simulink model "sampleModel188"  (R2021b)
settings: Solver=VariableStepAuto  StartTime=0.0  StopTime=10.0  RelTol=1e-3
libraries: simulink x11, slpidlib x1
settings Model: Creator=user  LastModifiedBy=user

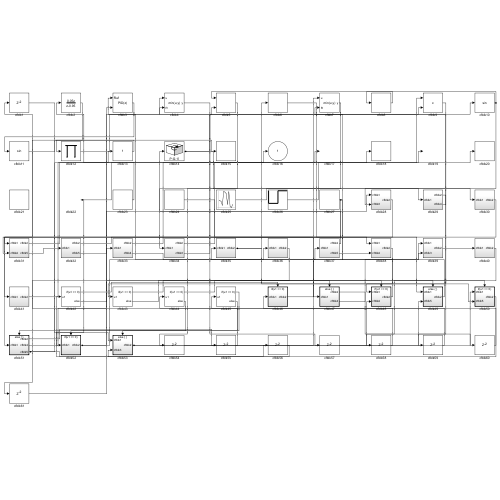
[thumbnail: Simulink's stored preview of the top-level diagram]
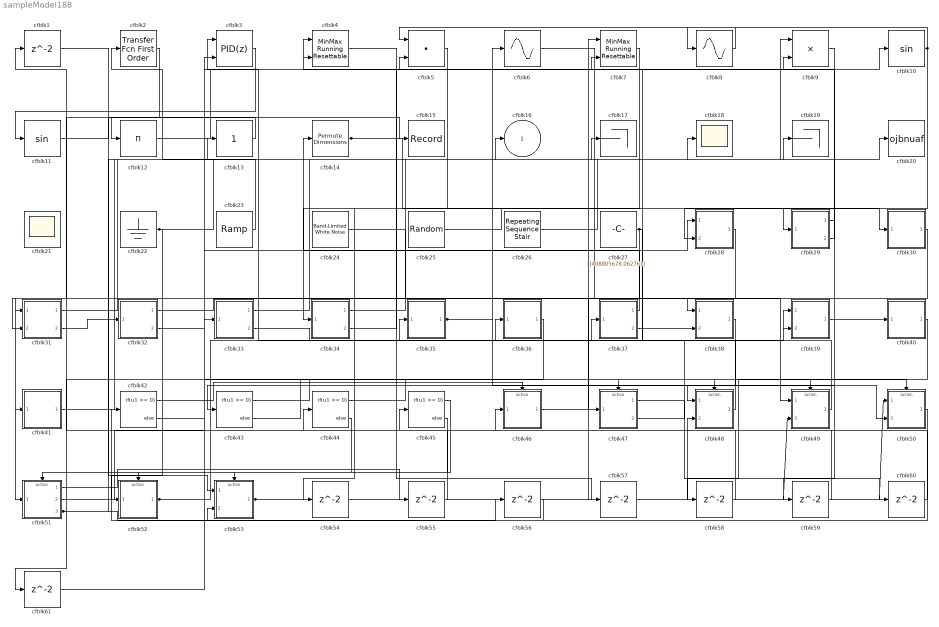
== system sampleModel188 ==
  cfblk{1,54..61} (9 alike) : Delay  SampleTime=1
  cfblk10 : Trigonometry
  cfblk11 : Trigonometry
  cfblk12 : Product  Inputs=*
  cfblk13 : simulink/Math Operations/Slider Gain  gain=1  low=0  high=2
  cfblk14 : PermuteDimensions
  cfblk15 : Record  FileSettingsInternal="{\"entries\":[{\"content\":{\"excelSettings\":{\"content\":{},\"type\":\"Streamout.ExcelSettings\"}},\"type\":\"Streamout.FileSettingStorage\",\"uuid\":\"ca993f84-a60c-403e-8350-93dc5c48e853\"}],\"packageUris\":[\"http://schema.mathworks.com/mf0/streamout_blocks/R2020a\"],\"version\":\"1.0\"}"  SignalsInternal="{\"entries\":[{\"content\":{\"signals\":[{\"content\":{\"blockPath\":[\"sampleModel188/cfblk15\"],\"channel\":[],\"dimensions\":[1,1],\"domain\":\"sampleModel188/cfblk15\",\"lineColor\":\"#139fff\",\"plots\":[1],\"port\":1,\"sid\":[\"\"],\"signalID\":7064,\"signalName\":\"cfblk11\"},\"type\":\"RecordBlkView.Signal\",\"uuid\":\"ba3ac5e5-cf71-48a5-8aa6-1fcd734a01e5\"}]},\"type\":\"RecordBlkView.InputSignals\",\"uuid\":\"2d8e7e94-0d17-40cb-8f9e-080a064f809d\"}],\"packageUris\":[\"http://schema.mathworks.com/mf0/streamout_blocks/R2020a\"],\"version\":\"1.0\"}"  VisualizationBindings="{\"sparklinesplugin\":{\"info\":[{\"bindingParametersList\":[],\"subplotID\":1}]}}"
  cfblk17 : Terminator
  cfblk18 : Scope
  cfblk19 : Terminator
  cfblk2 : simulink/Discrete/Transfer Fcn First Order  PoleZ=0.95  ICPrevOutput=0.0  DoSatur=off
  cfblk20 : ToWorkspace  VariableName=ojbnuaf  SaveFormat=Timeseries  SampleTime=-1
  cfblk21 : Scope
      settings: Floating=on
  cfblk22 : Ground
  cfblk23 : simulink/Sources/Ramp  slope=[6918.058367]  start=[43.830131]  InitialOutput=[-707195.429507]
  cfblk24 : simulink/Sources/Band-Limited White Noise  Cov=[2157080440.505384]  Ts=0.1  seed=[4930132520.000000]
  cfblk25 : RandomNumber  Mean=[-27753.868403]  Variance=[17619.578113]  Seed=[28560651.000000]  SampleTime=0.1
  cfblk26 : simulink/Sources/Repeating Sequence Stair  OutValues=[-496034706.787339, -122048597.583753]  tsamp=-1  OutMin=[]  OutMax=[]  OutDataTypeStr=double  OutputDataTypeScalingMode=double  OutDataType=fixdt(0,8)  ConRadixGroup=Best Precision: Vector-wise  OutScaling=2^-12
  cfblk27 : Constant  Value=[408805678.062761]  SampleTime=1
  cfblk28 : Subsystem
  cfblk29 : Subsystem
  cfblk3 : slpidlib/PID Controller (2DOF)  Controller=PID  Form=Parallel  TimeDomain=Discrete-time  UseExternalTs=off  SampleTime=1  IntegratorMethod=Forward Euler  FilterMethod=Forward Euler  ControllerParametersSource=internal  P=1  I=1  D=0  UseFilter=on  N=100  b=1  c=1  TunerSelectOption=Transfer Function Based (PID Tuner App)  InitialConditionSource=internal  InitialConditionForIntegrator=0  InitialConditionForFilter=0  DifferentiatorICPrevScaledInput=0  ExternalReset=none  TrackingMode=off  Kt=1  LimitOutput=off  SatLimitsSource=internal  UpperSaturationLimit=inf  LowerSaturationLimit=-inf  LinearizeAsGain=off  AntiWindupMode=none  Kb=1  POutMin=[]  POutMax=[]  IOutMin=[]  IOutMax=[]  DOutMin=[]  DOutMax=[]  NOutMin=[]  NOutMax=[]  bOutMin=[]  bOutMax=[]  cOutMin=[]  cOutMax=[]  SumOutMin=[]  SumOutMax=[]  SaturationOutMin=[]  SaturationOutMax=[]  PParamMin=[]  PParamMax=[]  IParamMin=[]  IParamMax=[]  DParamMin=[]  DParamMax=[]  NParamMin=[]  NParamMax=[]  bParamMin=[]  bParamMax=[]  cParamMin=[]  cParamMax=[]  KbParamMin=[]  KbParamMax=[]  KtParamMin=[]  KtParamMax=[]  KbOutMin=[]  KbOutMax=[]  KtOutMin=[]  KtOutMax=[]  IntegratorOutMin=[]  IntegratorOutMax=[]  FilterOutMin=[]  FilterOutMax=[]  SumI1OutMin=[]  SumI1OutMax=[]  SumI2OutMin=[]  SumI2OutMax=[]  SumI3OutMin=[]  SumI3OutMax=[]  SumI4OutMin=[]  SumI4OutMax=[]  SumDOutMin=[]  SumDOutMax=[]  Sum1OutMin=[]  Sum1OutMax=[]  Sum2OutMin=[]  Sum2OutMax=[]  Sum3OutMin=[]  Sum3OutMax=[]  DifferentiatorOutMin=[]  DifferentiatorOutMax=[]  FilterDiffOutCoefMin=[]  FilterDiffOutCoefMax=[]  ReciprocalOutMin=[]  ReciprocalOutMax=[]  SumDenOutMin=[]  SumDenOutMax=[]  SumNumOutMin=[]  SumNumOutMax=[]  DivideOutMin=[]  DivideOutMax=[]  UdiffTsProdOutMin=[]  UdiffTsProdOutMax=[]  NTsProdOutMin=[]  NTsProdOutMax=[]  UintegralTsProdOutMin=[]  UintegralTsProdOutMax=[]  UngainTsProdOutMin=[]  UngainTsProdOutMax=[]  IntegratorContinuousStateAttributes=''  IntegratorStateMustResolveToSignalObject=off  IntegratorRTWStateStorageClass=Auto  FilterContinuousStateAttributes=''  FilterStateMustResolveToSignalObject=off  FilterRTWStateStorageClass=Auto  ParallelPVariant=InternalParameters  IdealPVariant=Disabled  IVariant=InternalParameters  DVariant=InternalParameters  bVariant=InternalParameters  cVariant=InternalParameters  IntegratorVariant=Discrete  SatVariant=Disabled  AWVariant=Passthrough  PCopyVariant=Disabled  TRVariant=Disabled  FdbkBlocksVariant=Forward  IdealPFdbkVariant=Disabled  SatFdbkVariant=Disabled  DerivativeFilterVariant=ForwardEulerFilter  NVariant=InternalParameters  NCopyVariant=Disabled  FilterICVariant=InternalICsFilter  IntegratorICVariant=InternalICs  ExternalResetVariant=Disabled  TRSumVariant=Passthrough  SumFdbkVariant=Disabled  SumVariant=Sum_PID  TsampFilterVariant=InternalTs  TsampNgainVariant=Passthrough  TsampIntegralVariant=Passthrough  ExternalSaturationOutDataTypeStr=Inherit: Same as second input
      settings: SourceProductBaseCode=SL
  cfblk30 : Subsystem
  cfblk31 : Subsystem
  cfblk32 : Subsystem
  cfblk33 : Subsystem
  cfblk34 : Subsystem
  cfblk35 : Subsystem
  cfblk36 : Subsystem
  cfblk37 : Subsystem
  cfblk38 : Subsystem
  cfblk39 : Subsystem
  cfblk4 : simulink/Math Operations/MinMax Running Resettable  Function=min  vinit=0.0
  cfblk40 : Subsystem
  cfblk41 : Subsystem
  cfblk{42..45} (4 alike) : If  IfExpression=u1 >= 0  SampleTime=1
  cfblk46 : Subsystem  TreatAsAtomicUnit=on
  cfblk47 : Subsystem  TreatAsAtomicUnit=on
  cfblk48 : Subsystem  TreatAsAtomicUnit=on
  cfblk49 : Subsystem  TreatAsAtomicUnit=on
  cfblk5 : DotProduct  InputSameDT=on  OutDataTypeStr=Inherit: Inherit via internal rule
  cfblk50 : Subsystem  TreatAsAtomicUnit=on
  cfblk51 : Subsystem  TreatAsAtomicUnit=on
  cfblk52 : Subsystem  TreatAsAtomicUnit=on
  cfblk53 : Subsystem  TreatAsAtomicUnit=on
  cfblk6 : Sin  TimeSource=Use external signal  SampleTime=0
  cfblk7 : simulink/Math Operations/MinMax Running Resettable  Function=min  vinit=0.0
  cfblk8 : Sin  TimeSource=Use external signal  SampleTime=0
  cfblk9 : Product
  cfblk16 : Outport
  wires:
  cfblk29/1(cfblk2) -> cfblk48/1(cfblk1)
  cfblk41/1(cfblk2) -> cfblk19/1
  cfblk13/1 -> cfblk12/1
  cfblk3/1 -> cfblk11/1
  cfblk37/1(cfblk2) -> cfblk14/1
  cfblk27/1 -> cfblk35/1(cfblk1), cfblk31/2(cfblk4)
  cfblk12/1 -> cfblk4/1
  cfblk7/1 -> cfblk34/1(cfblk1)
  cfblk52/1(cfblk2) -> cfblk37/1(cfblk1), cfblk5/2
  cfblk33/1(cfblk2) -> cfblk16/1
  cfblk38/1(cfblk2) -> cfblk43/1
  cfblk26/1 -> cfblk18/1
  cfblk24/1 -> cfblk47/1(cfblk1)
  cfblk14/1 -> cfblk29/1(cfblk1), cfblk9/2
  cfblk35/1(cfblk2) -> cfblk6/1, cfblk50/2(cfblk5)
  cfblk25/1 -> cfblk30/1(cfblk1)
  cfblk33/2(cfblk4) -> cfblk36/1(cfblk1)
  cfblk23/1 -> cfblk2/1
  cfblk28/1(cfblk2) -> cfblk51/1(cfblk1)
  cfblk47/2(cfblk4) -> cfblk39/1(cfblk1)
  cfblk46/1(cfblk2) -> cfblk39/2(cfblk3)
  cfblk6/1 -> cfblk49/1(cfblk1)
  cfblk31/1(cfblk2) -> cfblk20/1
  cfblk29/2(cfblk4) -> cfblk4/2
  cfblk34/1(cfblk2) -> cfblk17/1
  cfblk32/1(cfblk2) -> cfblk38/1(cfblk1)
  cfblk10/1 -> cfblk8/1, cfblk28/2(cfblk3)
  cfblk50/1(cfblk2) -> cfblk42/1
  cfblk31/2(cfblk5) -> cfblk32/1(cfblk1)
  cfblk48/1(cfblk2) -> cfblk3/1
  cfblk11/1 -> cfblk15/1
  cfblk1/1 -> cfblk53/1(cfblk1)
  cfblk37/2(cfblk5) -> cfblk38/2(cfblk4)
  cfblk53/1(cfblk2) -> cfblk49/2(cfblk5), cfblk50/1(cfblk1)
  cfblk34/2(cfblk3) -> cfblk10/1
  cfblk30/1(cfblk2) -> cfblk41/1(cfblk1)
  cfblk49/1(cfblk2) -> cfblk7/2
  cfblk39/1(cfblk2) -> cfblk40/1(cfblk1)
  cfblk22/1 -> cfblk9/1, cfblk52/1(cfblk1)
  cfblk51/2(cfblk4) -> cfblk3/2
  cfblk8/1 -> cfblk5/1
  cfblk2/1 -> cfblk31/1(cfblk1)
  cfblk32/2(cfblk5) -> cfblk28/1(cfblk1)
  cfblk51/3(cfblk5) -> cfblk13/1, cfblk56/1
  cfblk42/1 -> cfblk46/Action
  cfblk42/2 -> cfblk47/Action
  cfblk43/1 -> cfblk48/Action
  cfblk43/2 -> cfblk49/Action
  cfblk44/1 -> cfblk50/Action
  cfblk44/2 -> cfblk51/Action
  cfblk45/1 -> cfblk52/Action
  cfblk45/2 -> cfblk53/Action
  cfblk5/1 -> cfblk54/1
  cfblk54/1 -> cfblk7/1
  cfblk51/1(cfblk2) -> cfblk55/1
  cfblk55/1 -> cfblk1/1
  cfblk56/1 -> cfblk53/2(cfblk3)
  cfblk4/1 -> cfblk57/1
  cfblk57/1 -> cfblk48/2(cfblk4)
  cfblk40/1(cfblk2) -> cfblk58/1
  cfblk58/1 -> cfblk46/1(cfblk1)
  cfblk9/1 -> cfblk59/1
  cfblk59/1 -> cfblk44/1
  cfblk47/1(cfblk2) -> cfblk60/1
  cfblk60/1 -> cfblk45/1
  cfblk36/1(cfblk2) -> cfblk61/1
  cfblk61/1 -> cfblk33/1(cfblk1)

== system sampleModel188/cfblk28 ==
  cfblk1 : Inport
  cfblk3 : Inport  Port=2
  cfblk2 : Outport
  wires:
  cfblk1/1 -> cfblk2/1

== system sampleModel188/cfblk29 ==
  cfblk1 : Inport
  cfblk3 : Gain  Gain=[-623215974.272057]
  cfblk2 : Outport
  cfblk4 : Outport  Port=2
  wires:
  cfblk1/1 -> cfblk4/1, cfblk3/1
  cfblk3/1 -> cfblk2/1

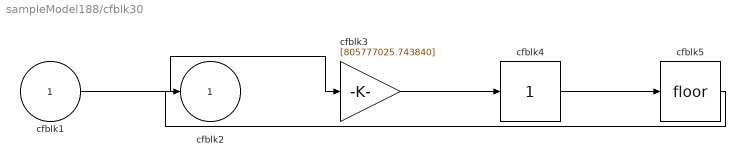
== system sampleModel188/cfblk30 ==
  cfblk1 : Inport
  cfblk3 : Gain  Gain=[805777025.743840]
  cfblk4 : simulink/Math Operations/Slider Gain  gain=1  low=0  high=2
  cfblk5 : Rounding
  cfblk2 : Outport
  wires:
  cfblk1/1 -> cfblk3/1
  cfblk3/1 -> cfblk4/1
  cfblk4/1 -> cfblk5/1
  cfblk5/1 -> cfblk2/1

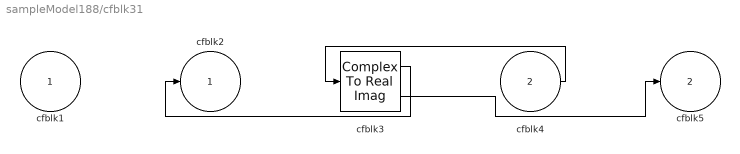
== system sampleModel188/cfblk31 ==
  cfblk1 : Inport
  cfblk4 : Inport  Port=2
  cfblk3 : ComplexToRealImag
  cfblk2 : Outport
  cfblk5 : Outport  Port=2
  wires:
  cfblk4/1 -> cfblk3/1
  cfblk3/1 -> cfblk2/1
  cfblk3/2 -> cfblk5/1

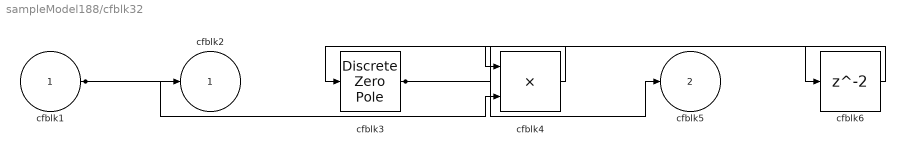
== system sampleModel188/cfblk32 ==
  cfblk1 : Inport
  cfblk3 : DiscreteZeroPole  Poles=[0 0.5]  Gain=1
  cfblk4 : Product  Inputs=**
  cfblk6 : Delay  SampleTime=1
  cfblk2 : Outport
  cfblk5 : Outport  Port=2
  wires:
  cfblk1/1 -> cfblk2/1, cfblk4/2
  cfblk3/1 -> cfblk5/1, cfblk6/1
  cfblk4/1 -> cfblk3/1
  cfblk6/1 -> cfblk4/1

== system sampleModel188/cfblk33 ==
  cfblk1 : Inport
  cfblk3 : ComplexToMagnitudeAngle
  cfblk2 : Outport
  cfblk4 : Outport  Port=2
  wires:
  cfblk3/1 -> cfblk2/1
  cfblk1/1 -> cfblk4/1, cfblk3/1

== system sampleModel188/cfblk34 ==
  cfblk1 : Inport
  cfblk2 : Outport
  cfblk3 : Outport  Port=2
  wires:
  cfblk1/1 -> cfblk2/1, cfblk3/1

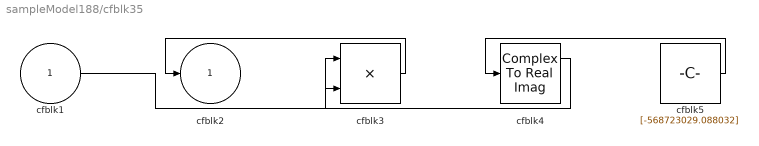
== system sampleModel188/cfblk35 ==
  cfblk1 : Inport
  cfblk3 : Product  Inputs=**
  cfblk4 : ComplexToRealImag
  cfblk5 : Constant  Value=[-568723029.088032]  SampleTime=1
  cfblk2 : Outport
  wires:
  cfblk5/1 -> cfblk4/1
  cfblk3/1 -> cfblk2/1
  cfblk1/1 -> cfblk3/1
  cfblk4/1 -> cfblk3/2

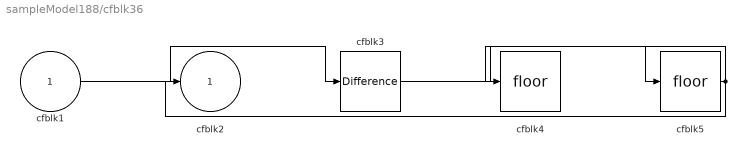
== system sampleModel188/cfblk36 ==
  cfblk1 : Inport
  cfblk3 : simulink/Discrete/Difference  ICPrevInput=0.0  OutMin=[]  OutMax=[]  OutDataTypeStr=Inherit: Inherit via back propagation  OutDataType=fixdt(1, 16)  OutScaling=2^-10  DoSatur=off
  cfblk4 : Rounding
  cfblk5 : Rounding
  cfblk2 : Outport
  wires:
  cfblk3/1 -> cfblk5/1
  cfblk1/1 -> cfblk3/1
  cfblk5/1 -> cfblk2/1, cfblk4/1

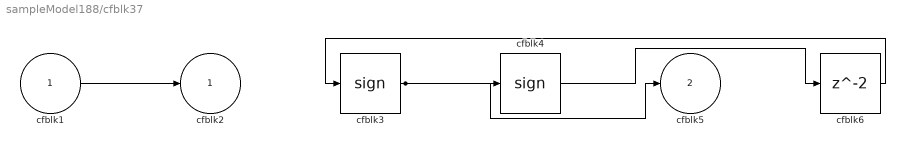
== system sampleModel188/cfblk37 ==
  cfblk1 : Inport
  cfblk3 : Signum
  cfblk4 : Signum
  cfblk6 : Delay  SampleTime=1
  cfblk2 : Outport
  cfblk5 : Outport  Port=2
  wires:
  cfblk1/1 -> cfblk2/1
  cfblk3/1 -> cfblk5/1, cfblk4/1
  cfblk4/1 -> cfblk6/1
  cfblk6/1 -> cfblk3/1

== system sampleModel188/cfblk38 ==
  cfblk1 : Inport
  cfblk4 : Inport  Port=2
  cfblk3 : simulink/Discrete/Transfer Fcn Lead or Lag  PoleZ=0.95  ZeroZ=0.75  ICPrevOutput=0.0  ICPrevInput=0.0  DoSatur=off
      settings: SourceProductBaseCode=SL
  cfblk2 : Outport
  wires:
  cfblk4/1 -> cfblk3/1
  cfblk3/1 -> cfblk2/1

== system sampleModel188/cfblk39 ==
  cfblk1 : Inport
  cfblk3 : Inport  Port=2
  cfblk2 : Outport
  wires:
  cfblk1/1 -> cfblk2/1

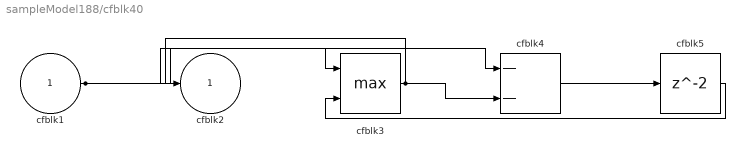
== system sampleModel188/cfblk40 ==
  cfblk1 : Inport
  cfblk3 : MinMax  Function=max  Inputs=2
  cfblk4 : Sum  Inputs=--
  cfblk5 : Delay  SampleTime=1
  cfblk2 : Outport
  wires:
  cfblk1/1 -> cfblk3/1, cfblk4/1
  cfblk3/1 -> cfblk2/1, cfblk4/2
  cfblk4/1 -> cfblk5/1
  cfblk5/1 -> cfblk3/2

== system sampleModel188/cfblk41 ==
  cfblk1 : Inport
  cfblk3 : Rounding
  cfblk4 : Product  Inputs=*
  cfblk2 : Outport
  wires:
  cfblk1/1 -> cfblk3/1
  cfblk4/1 -> cfblk2/1
  cfblk3/1 -> cfblk4/1

== system sampleModel188/cfblk46 ==
  cfblk1 : Inport
  Action Port : ActionPort  ActionPortLabel=if(u1 >= 0)
  cfblk3 : Delay  DelayLengthSource=Input port
      settings: InputPortMap=u0,p1
  cfblk4 : Product  Inputs=**
  cfblk2 : Outport
  wires:
  cfblk1/1 -> cfblk4/1, cfblk4/2
  cfblk4/1 -> cfblk3/1, cfblk3/2
  cfblk3/1 -> cfblk2/1

== system sampleModel188/cfblk47 ==
  cfblk1 : Inport
  Action Port : ActionPort  ActionPortLabel=else
  cfblk3 : Product
  cfblk2 : Outport
  cfblk4 : Outport  Port=2
  wires:
  cfblk1/1 -> cfblk2/1, cfblk3/1, cfblk3/2
  cfblk3/1 -> cfblk4/1

== system sampleModel188/cfblk48 ==
  cfblk1 : Inport
  cfblk4 : Inport  Port=2
  Action Port : ActionPort  ActionPortLabel=if(u1 >= 0)
  cfblk3 : Sum  Inputs=--
  cfblk2 : Outport
  wires:
  cfblk1/1 -> cfblk3/1
  cfblk4/1 -> cfblk3/2
  cfblk3/1 -> cfblk2/1

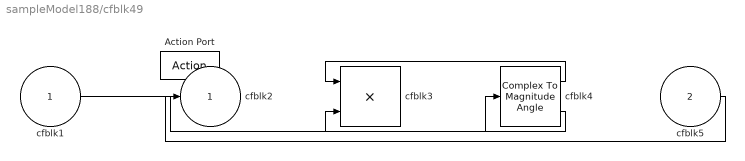
== system sampleModel188/cfblk49 ==
  cfblk1 : Inport
  cfblk5 : Inport  Port=2
  Action Port : ActionPort  ActionPortLabel=else
  cfblk3 : Product  Inputs=**
  cfblk4 : ComplexToMagnitudeAngle
  cfblk2 : Outport
  wires:
  cfblk1/1 -> cfblk4/1
  cfblk5/1 -> cfblk2/1
  cfblk4/1 -> cfblk3/1
  cfblk4/2 -> cfblk3/2

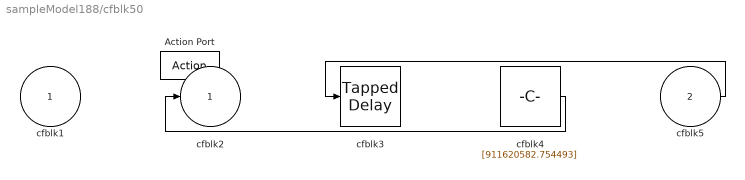
== system sampleModel188/cfblk50 ==
  cfblk1 : Inport
  cfblk5 : Inport  Port=2
  Action Port : ActionPort  ActionPortLabel=if(u1 >= 0)
  cfblk3 : simulink/Discrete/Tapped Delay  vinit=0.0  samptime=-1  NumDelays=1  DelayOrder=Oldest  includeCurrent=off
  cfblk4 : Constant  Value=[911620582.754493]  SampleTime=1
  cfblk2 : Outport
  wires:
  cfblk4/1 -> cfblk2/1
  cfblk5/1 -> cfblk3/1

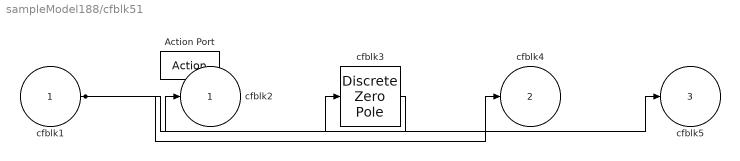
== system sampleModel188/cfblk51 ==
  cfblk1 : Inport
  Action Port : ActionPort  ActionPortLabel=else
  cfblk3 : DiscreteZeroPole  Poles=[0 0.5]  Gain=1  SampleTime=-1
  cfblk2 : Outport
  cfblk4 : Outport  Port=2
  cfblk5 : Outport  Port=3
  wires:
  cfblk3/1 -> cfblk2/1
  cfblk1/1 -> cfblk4/1, cfblk3/1, cfblk5/1

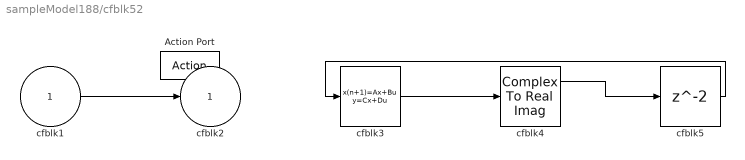
== system sampleModel188/cfblk52 ==
  cfblk1 : Inport
  Action Port : ActionPort  ActionPortLabel=if(u1 >= 0)
  cfblk3 : DiscreteStateSpace  SampleTime=-1
  cfblk4 : ComplexToRealImag
  cfblk5 : Delay
  cfblk2 : Outport
  wires:
  cfblk1/1 -> cfblk2/1
  cfblk3/1 -> cfblk4/1
  cfblk4/1 -> cfblk5/1
  cfblk5/1 -> cfblk3/1

== system sampleModel188/cfblk53 ==
  cfblk1 : Inport
  cfblk3 : Inport  Port=2
  Action Port : ActionPort  ActionPortLabel=else
  cfblk2 : Outport
  wires:
  cfblk3/1 -> cfblk2/1
